simulink model "D1_simuprueba"  (R2018a)
settings: Solver=VariableStepAuto  StartTime=0.0  StopTime=200  RelTol=1e-3
values from neighbouring files (symbols this model uses):
  TQQ = 2    [D_estimacion_planta.m]
  TSS = 1.2    [D_estimacion_planta.m]
undefined symbols (not defined in the file or in its folder): dQ, dS2, nQ, nS2
libraries: SignalEditorBlockLib x1
settings Model: Creator=quich  LastModifiedBy=glori

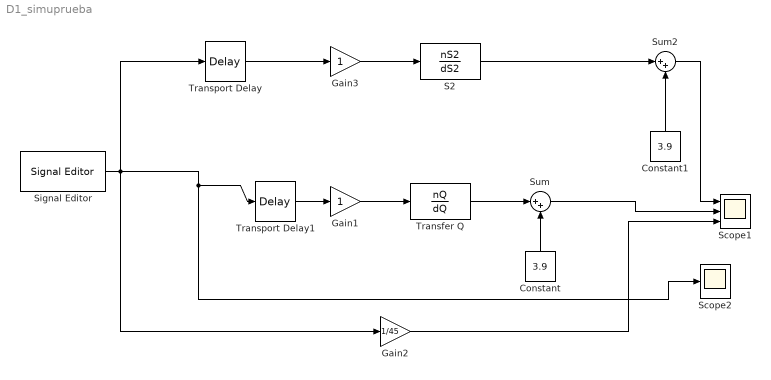
== system D1_simuprueba ==
  Constant : Constant  Value=3.9  SampleTime=0.055
  Constant1 : Constant  Value=3.9  SampleTime=0.055
  Gain1 : Gain
  Gain2 : Gain  Gain=1/45
  Gain3 : Gain
  S2 : TransferFcn  Numerator=nS2  Denominator=dS2
  Scope1 : Scope  NumInputPorts=3
  Scope2 : Scope
  Signal Editor : SignalEditorBlockLib/Signal Editor  FileName=escalon_5.mat  ActiveScenario=Scenario  ActiveSignal=Signal1  IsBus=off  OutputBusObjectStr=Bus: BusObject  SampleTime=0  Interpolate=off  ZeroCross=off  OutputAfterFinalValue=Setting to zero  Unit=inherit
  Sum : Sum  Inputs=|++
  Sum2 : Sum  Inputs=|++
  Transfer Q : TransferFcn  Numerator=nQ  Denominator=dQ
  Transport Delay : TransportDelay  DelayTime=TSS
  Transport Delay1 : TransportDelay  DelayTime=TQQ
  wires:
  Constant/1 -> Sum/2
  Gain1/1 -> Transfer Q/1
  Gain3/1 -> S2/1
  Signal Editor/1 -> Transport Delay1/1, Scope2/1, Transport Delay/1, Gain2/1
  Constant1/1 -> Sum2/2
  Transfer Q/1 -> Sum/1
  Sum/1 -> Scope1/2
  S2/1 -> Sum2/1
  Sum2/1 -> Scope1/1
  Gain2/1 -> Scope1/3
  Transport Delay/1 -> Gain3/1
  Transport Delay1/1 -> Gain1/1
